simulink model "Reaction_HW_start_2026"  (R2026a)
settings: Solver=FixedStepAuto
libraries: microbitledlib x5, microbitaccellib x2, microbitbuttonlib x2
settings Model: ExtModeTrigDuration=5  Creator=jaisohnk  LastModifiedBy=pinea
settings HardwareCC: ProdLargestAtomicInteger=Long  ProdLargestAtomicFloat=Double  ProdHWDeviceType=ARM Compatible->ARM Cortex
settings RTWCC: SystemTargetFile=ert.tlc  HardwareBoard=BBC micro:bit V2  TLCOptions=-aInlineSetEventsForThisBaseRateFcn=TLC_FALSE -aSuppressMultiTaskScheduler=TLC_FALSE -aRateBasedStepFcn=1  Toolchain=GNU Tools for ARM Embedded Processors  Description=Embedded Coder
settings ERTTargetCC: ExtModeTransport=3.0

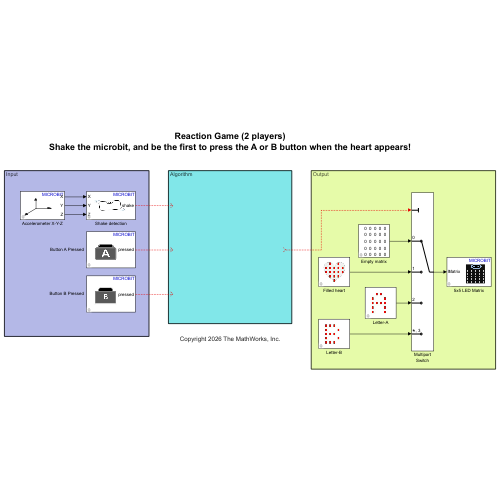
[thumbnail: Simulink's stored preview of the top-level diagram]
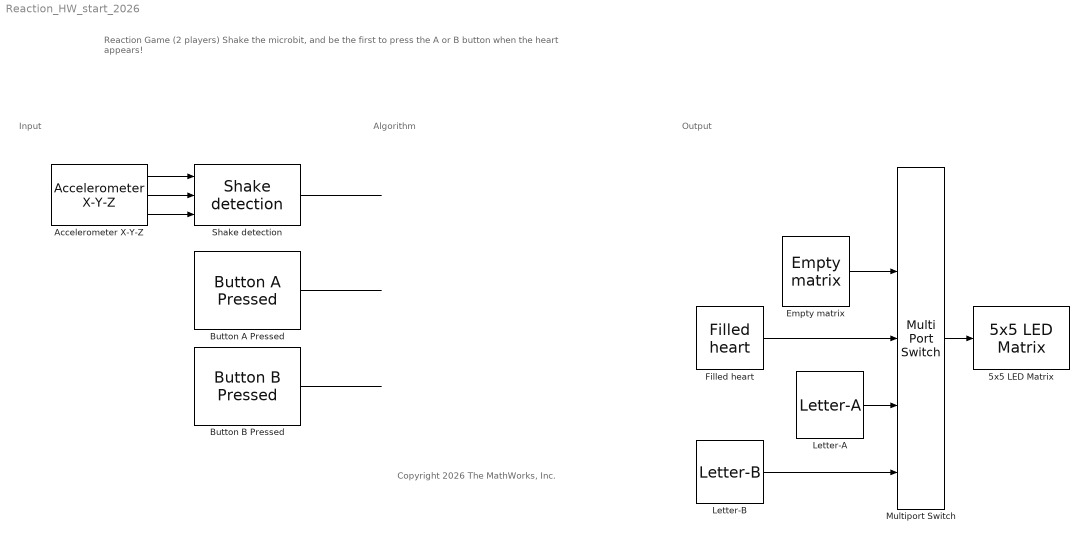
== system Reaction_HW_start_2026 ==
  note: Input
  note: Output
  note: Reaction Game (2 players)
      | Shake the microbit, and be the first to press the A or B button when the heart appears!
  note: Algorithm
  note: Copyright 2026 The MathWorks, Inc.
  5x5 LED Matrix : microbitledlib/5x5 LED Matrix  LED_mat=[0 1 1 1 0;1 0 1 0 1;1 1 0 1 1; 1 0 1 0 1;0 1 1 1 0]
  Accelerometer X-Y-Z : microbitaccellib/Accelerometer X-Y-Z  ODR=200Hz  Accelfullrange=-2g to +2g  SampleTime=0.1
  Button A Pressed : microbitbuttonlib/Button A Pressed  SampleTime=0.1
  Button B Pressed : microbitbuttonlib/Button B Pressed  SampleTime=0.1
  Empty matrix : microbitledlib/LED Images/Empty matrix  L00=off  L01=off  L02=off  L03=off  L04=off  L10=off  L11=off  L12=off  L13=off  L14=off  L20=off  L21=off  L22=off  L23=off  L24=off  L30=off  L31=off  L32=off  L33=off  L34=off  L40=off  L41=off  L42=off  L43=off  L44=off
  Filled heart : microbitledlib/LED Images/Filled heart
  Letter-A : microbitledlib/LED Images/Letter-A  L00=off  L01=on  L02=on  L03=off  L04=off  L10=on  L11=off  L12=off  L13=on  L14=off  L20=on  L21=on  L22=on  L23=on  L24=off  L30=on  L31=off  L32=off  L33=on  L34=off  L40=on  L41=off  L42=off  L43=on  L44=off
  Letter-B : microbitledlib/LED Images/Letter-B  L00=on  L01=on  L02=on  L03=off  L04=off  L10=on  L11=off  L12=off  L13=on  L14=off  L20=on  L21=on  L22=on  L23=off  L24=off  L30=on  L31=off  L32=off  L33=on  L34=off  L40=on  L41=on  L42=on  L43=off  L44=off
  Multiport Switch : MultiPortSwitch  DataPortOrder=Zero-based contiguous  Inputs=4  zeroidx=on  SaturateOnIntegerOverflow=off  InputSameDT=off
  Shake detection : microbitaccellib/Shake detection  sen=3
  wires:
  Accelerometer X-Y-Z/2 -> Shake detection/2
  Letter-A/1 -> Multiport Switch/4
  Button A Pressed/1 -> ?
  Accelerometer X-Y-Z/3 -> Shake detection/3
  Letter-B/1 -> Multiport Switch/5
  Accelerometer X-Y-Z/1 -> Shake detection/1
  Empty matrix/1 -> Multiport Switch/2
  Multiport Switch/1 -> 5x5 LED Matrix/1
  Shake detection/1 -> ?
  ? -> Multiport Switch/1
  Filled heart/1 -> Multiport Switch/3
  Button B Pressed/1 -> ?
